simulink model "Modelo_NL_Final"  (R2018a)
settings: Solver=VariableStepAuto  StartTime=0.0  StopTime=2500  RelTol=1e-3
values from neighbouring files (symbols this model uses):
  A = [xu,        xw*u0,         -u0*tan(aa0), -g*cos(tt0),     0 ... (first row only)    [long_ctes.m]    (also in modelo_L13_PD_lateral.m = [ybb yp+w0/u0 yr-1 g*cos(tt0)/u0 ; lbb lp lr 0 ; nbb np nr 0; real_servo_c_lateral.m = [ybb yp+w0/u0 yr-1 g*cos(tt0)/u0 0; lbb lp lr 0 0; nbb np nr)
  A_lat = [ybb yp+w0/u0 yr-1 g*cos(tt0)/u0 0; lbb lp lr 0 0; nbb np nr 0 0; 0 1 tan(tt0) 0 0; 0 0 1/cos(tt0) 0 0]    [lateral_ctes.m]
  B = [xde,         xdf ... (first row only)    [long_ctes.m]    (also in modelo_L13_PD_lateral.m = [0 Ydr ; Lda Ldr ; Nda Ndr ; 0 0]; real_servo_c_lateral.m = [0 Ydr ; Lda Ldr ; Nda Ndr ; 0 0 ; 0 0])
  B_lat = [0 Ydr ; Lda Ldr ; Nda Ndr ; 0 0 ; 0 0]    [lateral_ctes.m]
  C_lat = eye(5)    [lateral_ctes.m]
  Cc_lat = C_lat(2:1:4,:)    [lateral_ctes.m]
  Cy_lat = C_lat(1:4:5,:)    [lateral_ctes.m]
  D_lat = [0 0; 0 0; 0 0; 0 0; 0 0]    [lateral_ctes.m]
  deg = pi/180    (= 0.0174532925199)    [lateral_ctes.m]    (also in long_ctes.m; modelo_L13_PD_lateral.m; real_servo_c_lateral.m)
  demax = 28*deg    (= 0.488692190558)    [long_ctes.m]    (also in modelo_L13_PD_lateral.m = [+28 -21]; real_servo_c_lateral.m = [+28 -21])
  demin = -21*deg    (= -0.366519142919)    [long_ctes.m]
  inicial = [u0, aa0, 0, tt0, h0]    [long_ctes.m]
  Kc = [-0.0196 1.6622 -0.8045 -3.0813 -0.0000 0.9333]    [long_ctes.m]    (also in real_servo_c_lateral.m = k(:,2:1:4))
  Kc_lat = k_lat(:,2:1:4)    [lateral_ctes.m]
  Ky_lat = k_lat(:,1:4:5)    [lateral_ctes.m]
  pontos_T = pontos.'    [coordenadas2.m]
libraries: simulink x7, dspsigops x1
settings Model: Creator=tiagogomes  LastModifiedBy=tiagogomes
settings DataIOCC: ReturnWorkspaceOutputs=on
settings SFSimCC: SimUseLocalCustomCode=on
settings RTWCC: RTWUseLocalCustomCode=on

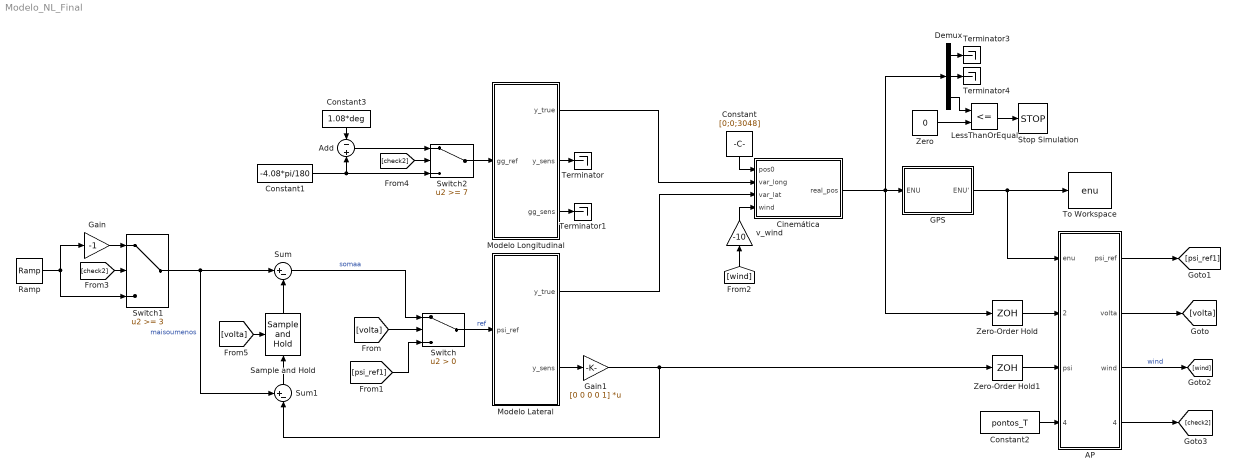
== system Modelo_NL_Final ==
  AP : MATLAB Function  TreatAsAtomicUnit=on
  Add : Sum  Inputs=-+
  Cinemática : Subsystem
  Constant : Constant  Value=[0;0;3048]
  Constant1 : Constant  Value=-4.08*pi/180
  Constant2 : Constant  Value=pontos_T
  Constant3 : Constant  Value=1.08*deg
  Demux : Demux  Outputs=3
  GPS : Subsystem
  Gain : Gain  Gain=-1
  Gain1 : Gain  Gain=[0 0 0 0 1]  Multiplication=Matrix(K*u)
  LessThanOrEqual : RelationalOperator  Operator=<=  OutDataTypeStr=boolean  RndMeth=Simplest
  Modelo Lateral : Subsystem
  Modelo Longitudinal : Subsystem  TreatAsAtomicUnit=on
  Ramp : simulink/Sources/Ramp  slope=-0.192  start=0  InitialOutput=0
  Sample and Hold : dspsigops/Sample and Hold  trig=Rising edge  initCond=0  latchinput=off
  Stop Simulation : Stop
  Sum : Sum  Inputs=|+-
  Sum1 : Sum  Inputs=+-|
  Switch : Switch  Criteria=u2 > Threshold
  Switch1 : Switch  Threshold=3
  Switch2 : Switch  Threshold=7
  Terminator{,1,3..4} (4 alike) : Terminator
  To Workspace : ToWorkspace  VariableName=enu  SampleTime=-1
      settings: Save2DSignal=2-D array (concatenate along first dimension)
  Zero : Constant  Value=0  OutDataTypeStr=Inherit: Inherit via back propagation
  Zero-Order Hold : ZeroOrderHold
  Zero-Order Hold1 : ZeroOrderHold
  v_wind : Gain  Gain=-10
  wires:
  Constant/1 -> Cinemática/1(pos0)
  Modelo Longitudinal/1(y_true) -> Cinemática/2(var_long)
  Modelo Lateral/1(y_true) -> Cinemática/3(var_lat)
  Constant1/1 -> Add/2, Switch2/3
  Modelo Longitudinal/2(y_sens) -> Terminator/1
  Modelo Longitudinal/3(gg_sens) -> Terminator1/1
  Cinemática/1(real_pos) -> Zero-Order Hold/1, Demux/1, GPS/1(ENU)
  GPS/1(ENU') -> AP/1(enu), To Workspace/1
  Constant2/1 -> AP/4(pontos_T)
  v_wind/1 -> Cinemática/4(wind)
  [volta] -> Switch/2
  AP/1(psi_ref) -> [psi_ref1]
  Switch/1 -> Modelo Lateral/1(psi_ref)  "ref"
  [psi_ref1] -> Switch/3
  Zero-Order Hold/1 -> AP/2(enu_real)
  AP/2(volta) -> [volta]
  AP/3(wind) -> [wind]  "wind"
  [wind] -> v_wind/1
  Gain/1 -> Switch1/1
  AP/4(check2) -> [check2]
  [check2] -> Switch1/2
  Zero/1 -> LessThanOrEqual/2
  Demux/3 -> LessThanOrEqual/1
  LessThanOrEqual/1 -> Stop Simulation/1
  Constant3/1 -> Add/1
  Switch2/1 -> Modelo Longitudinal/1(gg_ref)
  Add/1 -> Switch2/1
  [check2] -> Switch2/2
  Demux/1 -> Terminator3/1
  Demux/2 -> Terminator4/1
  [volta] -> Sample and Hold/Trigger
  Modelo Lateral/2(y_sens) -> Gain1/1
  Gain1/1 -> Sum1/2, Zero-Order Hold1/1
  Sample and Hold/1 -> Sum/2
  Ramp/1 -> Switch1/3, Gain/1
  Sum1/1 -> Sample and Hold/1
  Switch1/1 -> Sum1/1, Sum/1  "maisoumenos"
  Sum/1 -> Switch/1  "somaa"
  Zero-Order Hold1/1 -> AP/3(psi)

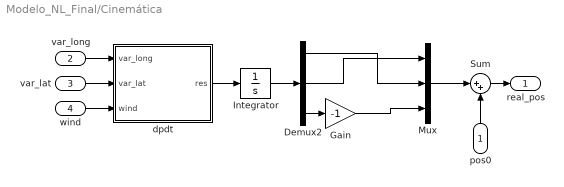
== system Modelo_NL_Final/Cinemática ==
  pos0 : Inport
  var_long : Inport  Port=2
  var_lat : Inport  Port=3
  wind : Inport  Port=4
  Demux2 : Demux  Outputs=3
  Gain : Gain  Gain=-1
  Integrator : Integrator
  Mux : Mux  Inputs=3
  Sum : Sum  Inputs=|++
  dpdt : MATLAB Function  TreatAsAtomicUnit=on
  real_pos : Outport
  wires:
  var_long/1 -> dpdt/1(var_long)
  wind/1 -> dpdt/3(wind)
  dpdt/1(res) -> Integrator/1
  Sum/1 -> real_pos/1
  var_lat/1 -> dpdt/2(var_lat)
  pos0/1 -> Sum/2
  Integrator/1 -> Demux2/1
  Demux2/1 -> Mux/2
  Mux/1 -> Sum/1
  Demux2/2 -> Mux/1
  Demux2/3 -> Gain/1
  Gain/1 -> Mux/3

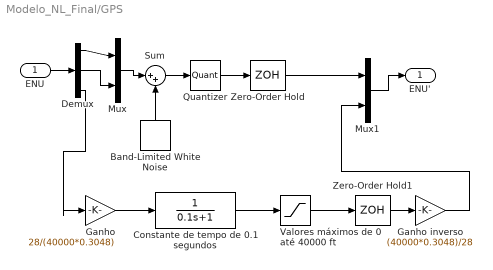
== system Modelo_NL_Final/GPS ==
  ENU : Inport
  Band-Limited White Noise : simulink/Sources/Band-Limited White Noise  Cov=16  Ts=1  seed=[23341]
  Constante de tempo de 0.1 segundos : TransferFcn  Denominator=[0.1 1]
  Demux : Demux  Outputs=3
  Ganho : Gain  Gain=28/(40000*0.3048)
  Ganho inverso : Gain  Gain=(40000*0.3048)/28
  Mux : Mux  Inputs=2
  Mux1 : Mux  Inputs=2
  Quantizer : Quantizer
  Sum : Sum  Inputs=|++
  Valores máximos de 0 até 40000 ft : Saturate  UpperLimit=28  LowerLimit=0
  Zero-Order Hold : ZeroOrderHold
  Zero-Order Hold1 : ZeroOrderHold
  ENU' : Outport
  wires:
  Sum/1 -> Quantizer/1
  Quantizer/1 -> Zero-Order Hold/1
  Band-Limited White Noise/1 -> Sum/2
  Ganho/1 -> Constante de tempo de 0.1 segundos/1
  Ganho inverso/1 -> Mux1/2
  Constante de tempo de 0.1 segundos/1 -> Valores máximos de 0 até 40000 ft/1
  ENU/1 -> Demux/1
  Demux/2 -> Mux/2
  Demux/1 -> Mux/1
  Mux/1 -> Sum/1
  Demux/3 -> Ganho/1
  Zero-Order Hold/1 -> Mux1/1
  Mux1/1 -> ENU'/1
  Valores máximos de 0 até 40000 ft/1 -> Zero-Order Hold1/1
  Zero-Order Hold1/1 -> Ganho inverso/1

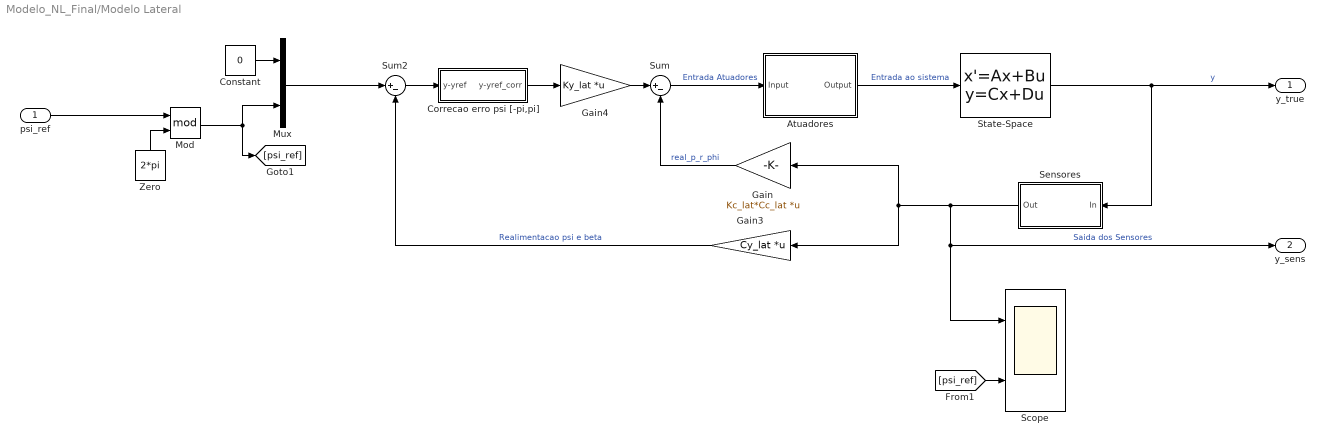
== system Modelo_NL_Final/Modelo Lateral ==
  psi_ref : Inport
  Atuadores : Subsystem
  Constant : Constant  Value=0
  Correcao erro psi [-pi,pi] : Subsystem
  Gain : Gain  Gain=Kc_lat*Cc_lat  Multiplication=Matrix(K*u)
  Gain3 : Gain  Gain=Cy_lat  Multiplication=Matrix(K*u)
  Gain4 : Gain  Gain=Ky_lat  Multiplication=Matrix(K*u)
  Mod : Math  Operator=mod  SaturateOnIntegerOverflow=on
  Mux : Mux  Inputs=2
  Scope : Scope  NumInputPorts=2
  Sensores : Subsystem
  State-Space : StateSpace  A=A_lat  B=B_lat  C=C_lat  D=D_lat  InitialCondition=[0 0 0 0 2.8254]  ContinuousStateAttributes={'beta','p','r','pranchamento','guinada'}
  Sum : Sum  Inputs=|+-
  Sum2 : Sum  Inputs=|+-
  Zero : Constant  Value=2*pi  OutDataTypeStr=Inherit: Inherit via back propagation
  y_true : Outport
  y_sens : Outport  Port=2
  wires:
  Constant/1 -> Mux/1
  Correcao erro psi [-pi,pi]/1(y-yref_corr) -> Gain4/1
  Mod/1 -> Mux/2, [psi_ref]
  State-Space/1 -> y_true/1, Sensores/1(In)  "y"
  Gain4/1 -> Sum/1
  Mux/1 -> Sum2/1
  Sensores/1(Out) -> Gain/1, Gain3/1, Scope/1, y_sens/1  "Saida dos Sensores"
  Gain/1 -> Sum/2  "real_p_r_phi"
  Atuadores/1(Output) -> State-Space/1  "Entrada ao sistema"
  [psi_ref] -> Scope/2
  Gain3/1 -> Sum2/2  "Realimentacao psi e beta"
  Sum/1 -> Atuadores/1(Input)  "Entrada Atuadores"
  Sum2/1 -> Correcao erro psi [-pi,pi]/1(y-yref)
  Zero/1 -> Mod/2
  psi_ref/1 -> Mod/1

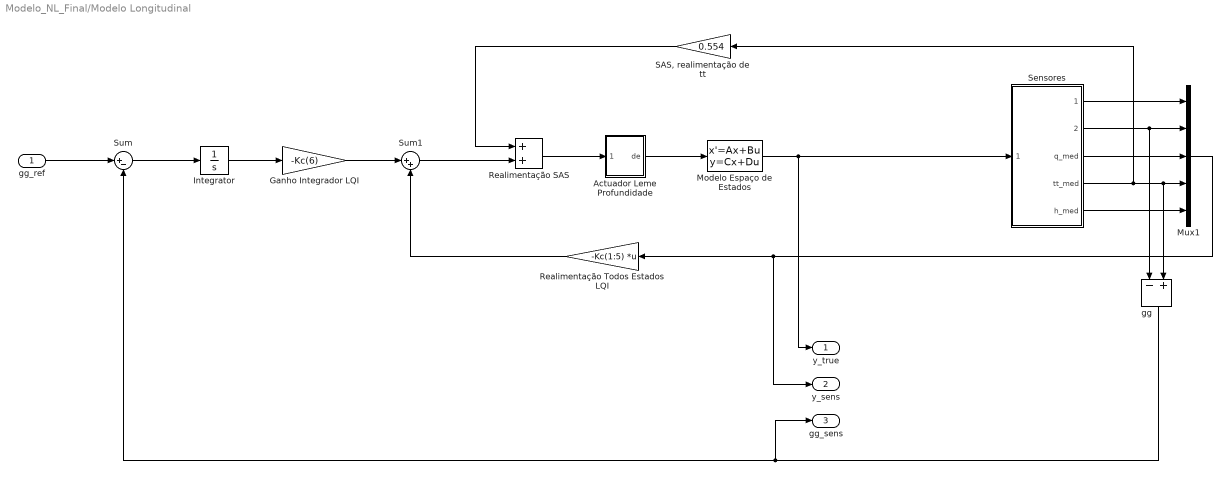
== system Modelo_NL_Final/Modelo Longitudinal ==
  gg_ref : Inport
  "Actuador Leme Profundidade " : Subsystem
  Ganho Integrador LQI : Gain  Gain=-Kc(6)
  Integrator : Integrator
  Modelo Espaço de Estados : StateSpace  A=A  B=B(:,1)  C=eye(5)  D=[0; 0; 0; 0; 0]  InitialCondition=inicial  ContinuousStateAttributes={'u', 'aa', 'q', 'tt', 'h'}
  Mux1 : Mux  Inputs=5
  Realimentação SAS : Sum
  Realimentação Todos Estados LQI : Gain  Gain=-Kc(1:5)  Multiplication=Matrix(K*u) (u vector)
  "SAS, realimentação de tt" : Gain  Gain=0.554
  Sensores : Subsystem
  Sum : Sum  Inputs=|+-
  Sum1 : Sum  Inputs=|++
  gg : Sum  Inputs=-+
  y_true : Outport
  y_sens : Outport  Port=2
  gg_sens : Outport  Port=3
  wires:
  gg_ref/1 -> Sum/1
  Sum/1 -> Integrator/1
  Integrator/1 -> Ganho Integrador LQI/1
  Ganho Integrador LQI/1 -> Sum1/1
  "Actuador Leme Profundidade "/1(de) -> Modelo Espaço de Estados/1
  "SAS, realimentação de tt"/1 -> Realimentação SAS/1
  Sum1/1 -> Realimentação SAS/2
  Realimentação Todos Estados LQI/1 -> Sum1/2
  Realimentação SAS/1 -> "Actuador Leme Profundidade "/1(de0)
  Modelo Espaço de Estados/1 -> Sensores/1(Estados), y_true/1
  Sensores/4(tt_med) -> gg/2, Mux1/4, "SAS, realimentação de tt"/1
  Sensores/1(TAS_med) -> Mux1/1
  Sensores/2(aa_med) -> gg/1, Mux1/2
  Sensores/3(q_med) -> Mux1/3
  Sensores/5(h_med) -> Mux1/5
  Mux1/1 -> y_sens/1, Realimentação Todos Estados LQI/1
  gg/1 -> gg_sens/1, Sum/2

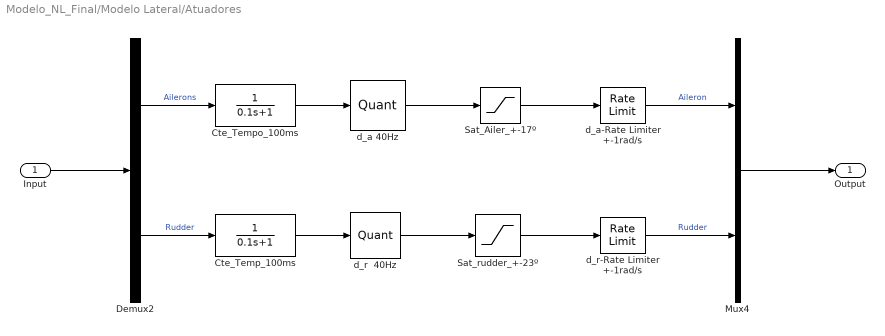
== system Modelo_NL_Final/Modelo Lateral/Atuadores ==
  Input : Inport
  Cte_Temp_100ms : TransferFcn  Denominator=[0.1 1]
  Cte_Tempo_100ms : TransferFcn  Denominator=[0.1 1]
  Demux2 : Demux  Outputs=2
  Mux4 : Mux  Inputs=2
  Sat_Ailer_+-17º : Saturate  UpperLimit=17*deg  LowerLimit=-17*deg
  Sat_rudder_+-23º : Saturate  UpperLimit=23*deg  LowerLimit=-23*deg
  d_a 40Hz : Quantizer  QuantizationInterval=1/40
  d_a-Rate Limiter +-1rad/s : RateLimiter  SampleTimeMode=inherited
  d_r  40Hz : Quantizer  QuantizationInterval=1/40
  d_r-Rate Limiter +-1rad/s : RateLimiter  SampleTimeMode=inherited
  Output : Outport
  wires:
  d_a 40Hz/1 -> Sat_Ailer_+-17º/1
  Input/1 -> Demux2/1
  Sat_rudder_+-23º/1 -> d_r-Rate Limiter +-1rad/s/1
  Mux4/1 -> Output/1
  Cte_Temp_100ms/1 -> d_r  40Hz/1
  d_r  40Hz/1 -> Sat_rudder_+-23º/1
  d_r-Rate Limiter +-1rad/s/1 -> Mux4/2  "Rudder"
  Demux2/2 -> Cte_Temp_100ms/1  "Rudder"
  d_a-Rate Limiter +-1rad/s/1 -> Mux4/1  "Aileron"
  Demux2/1 -> Cte_Tempo_100ms/1  "Ailerons"
  Cte_Tempo_100ms/1 -> d_a 40Hz/1
  Sat_Ailer_+-17º/1 -> d_a-Rate Limiter +-1rad/s/1

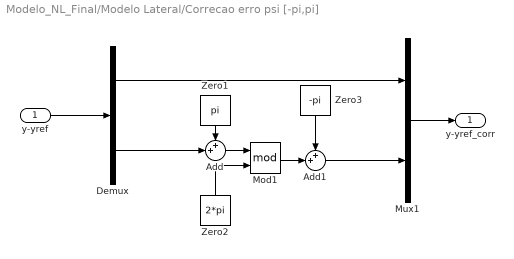
== system Modelo_NL_Final/Modelo Lateral/Correcao erro psi [-pi,pi] ==
  y-yref : Inport
  Add : Sum  Inputs=++|
  Add1 : Sum  Inputs=++|
  Demux : Demux  Outputs=2
  Mod1 : Math  Operator=mod  SaturateOnIntegerOverflow=on
  Mux1 : Mux  Inputs=2
  Zero1 : Constant  Value=pi  OutDataTypeStr=Inherit: Inherit via back propagation
  Zero2 : Constant  Value=2*pi  OutDataTypeStr=Inherit: Inherit via back propagation
  Zero3 : Constant  Value=-pi  OutDataTypeStr=Inherit: Inherit via back propagation
  y-yref_corr : Outport
  wires:
  Zero1/1 -> Add/1
  Zero3/1 -> Add1/1
  Zero2/1 -> Mod1/2
  Mod1/1 -> Add1/2
  y-yref/1 -> Demux/1
  Add/1 -> Mod1/1
  Mux1/1 -> y-yref_corr/1
  Add1/1 -> Mux1/2
  Demux/2 -> Add/2
  Demux/1 -> Mux1/1

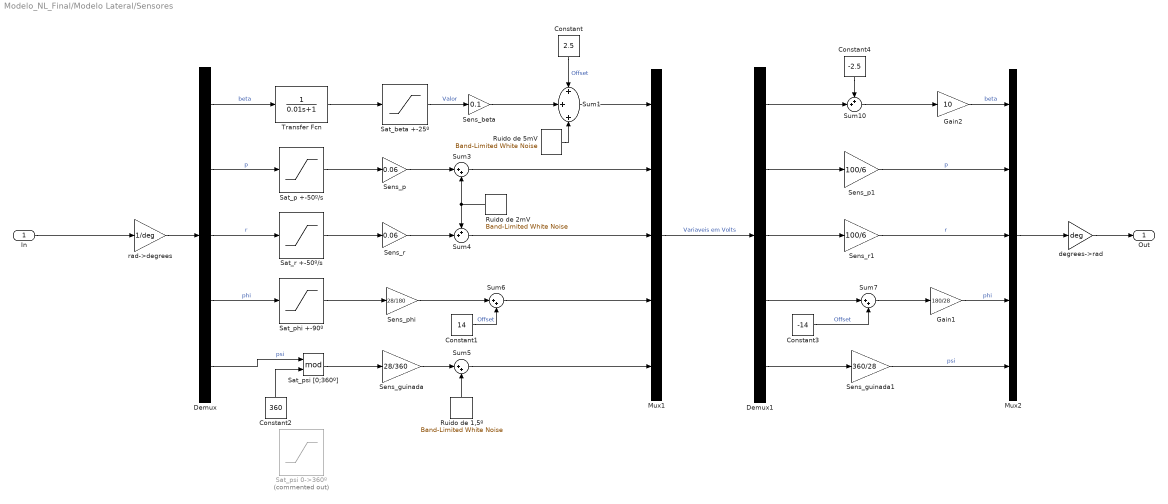
== system Modelo_NL_Final/Modelo Lateral/Sensores ==
  In : Inport
  Constant : Constant  Value=2.5
  Constant1 : Constant  Value=14
  Constant2 : Constant  Value=360
  Constant3 : Constant  Value=-14
  Constant4 : Constant  Value=-2.5
  Demux : Demux  Outputs=5
  Demux1 : Demux  Outputs=5
  Gain1 : Gain  Gain=180/28
  Gain2 : Gain  Gain=10
  Mux1 : Mux  Inputs=5
  Mux2 : Mux  Inputs=5
  Ruido de 1,5º : simulink/Sources/Band-Limited White Noise  Cov=[(1.5*28/360)^2/40]  Ts=1/40  seed=[23341]
  Ruido de 2mV : simulink/Sources/Band-Limited White Noise  Cov=[(0.002)^2/40]  Ts=1/40  seed=[23341]
  Ruido de 5mV : simulink/Sources/Band-Limited White Noise  Cov=[(0.005)^2/40]  Ts=1/40  seed=[23341]
  Sat_beta +-25º : Saturate  UpperLimit=+25  LowerLimit=-25
  Sat_p +-50º/s : Saturate  UpperLimit=+50  LowerLimit=-50
  Sat_phi +-90º : Saturate  UpperLimit=+90  LowerLimit=-90
  Sat_psi 0->360º : Saturate  Commented=on  UpperLimit=360  LowerLimit=-360
  Sat_psi [0;360º] : Math  Operator=mod  SaturateOnIntegerOverflow=on
  Sat_r +-50º/s : Saturate  UpperLimit=+50  LowerLimit=-50
  Sens_beta : Gain  Gain=0.1
  Sens_guinada : Gain  Gain=28/360
  Sens_guinada1 : Gain  Gain=360/28
  Sens_p : Gain  Gain=0.06
  Sens_p1 : Gain  Gain=100/6
  Sens_phi : Gain  Gain=28/180
  Sens_r : Gain  Gain=0.06
  Sens_r1 : Gain  Gain=100/6
  Sum1 : Sum  Inputs=+++
  Sum10 : Sum  Inputs=++|
  Sum{3,5..7} (4 alike) : Sum  Inputs=|++
  Sum4 : Sum  Inputs=++|
  Transfer Fcn : TransferFcn  Denominator=[0.01 1]
  degrees->rad : Gain  Gain=deg
  rad->degrees : Gain  Gain=1/deg
  Out : Outport
  wires:
  Sens_guinada/1 -> Sum5/1
  Demux1/4 -> Sum7/1
  Gain2/1 -> Mux2/1  "beta"
  Sens_phi/1 -> Sum6/1
  Demux1/5 -> Sens_guinada1/1
  Sat_p +-50º/s/1 -> Sens_p/1
  Sum6/1 -> Mux1/4
  Sens_p1/1 -> Mux2/2  "p"
  Constant1/1 -> Sum6/2  "Offset"
  Sens_beta/1 -> Sum1/2
  Ruido de 5mV/1 -> Sum1/3
  Sens_r1/1 -> Mux2/3  "r"
  In/1 -> rad->degrees/1
  Sat_beta +-25º/1 -> Sens_beta/1  "Valor"
  Constant3/1 -> Sum7/2  "Offset"
  degrees->rad/1 -> Out/1
  Sum4/1 -> Mux1/3
  Demux/4 -> Sat_phi +-90º/1  "phi"
  Sum7/1 -> Gain1/1
  Sens_r/1 -> Sum4/2
  Sum10/1 -> Gain2/1
  Gain1/1 -> Mux2/4  "phi"
  rad->degrees/1 -> Demux/1
  Mux1/1 -> Demux1/1  "Variaveis em Volts"
  Sens_guinada1/1 -> Mux2/5  "psi"
  Sum5/1 -> Mux1/5
  Sat_phi +-90º/1 -> Sens_phi/1
  Demux/2 -> Sat_p +-50º/s/1  "p"
  Sum1/1 -> Mux1/1
  Demux/3 -> Sat_r +-50º/s/1  "r"
  Ruido de 1,5º/1 -> Sum5/2
  Ruido de 2mV/1 -> Sum3/2, Sum4/1
  Mux2/1 -> degrees->rad/1
  Sens_p/1 -> Sum3/1
  Sum3/1 -> Mux1/2
  Constant/1 -> Sum1/1  "Offset"
  Sat_r +-50º/s/1 -> Sens_r/1
  Demux1/3 -> Sens_r1/1
  Demux1/2 -> Sens_p1/1
  Demux/1 -> Transfer Fcn/1  "beta"
  Transfer Fcn/1 -> Sat_beta +-25º/1
  Demux1/1 -> Sum10/2
  Constant4/1 -> Sum10/1
  Demux/5 -> Sat_psi [0;360º]/1  "psi"
  Sat_psi [0;360º]/1 -> Sens_guinada/1
  Constant2/1 -> Sat_psi [0;360º]/2

== system Modelo_NL_Final/Modelo Longitudinal/Actuador Leme Profundidade  ==
  de0 : Inport
  Amostragem 40Hz : ZeroOrderHold  SampleTime=1/40
  Constante de tempo de 0.1 segundos : TransferFcn  Denominator=[0.1 1]
  Deflexões máximas +28º / -21º : Saturate  UpperLimit=demax  LowerLimit=demin
  Velocidade deflexão máxima 1 rad/s : RateLimiter  SampleTimeMode=inherited
  de : Outport
  wires:
  de0/1 -> Constante de tempo de 0.1 segundos/1
  Constante de tempo de 0.1 segundos/1 -> Amostragem 40Hz/1
  Amostragem 40Hz/1 -> Deflexões máximas +28º / -21º/1
  Deflexões máximas +28º / -21º/1 -> Velocidade deflexão máxima 1 rad/s/1
  Velocidade deflexão máxima 1 rad/s/1 -> de/1

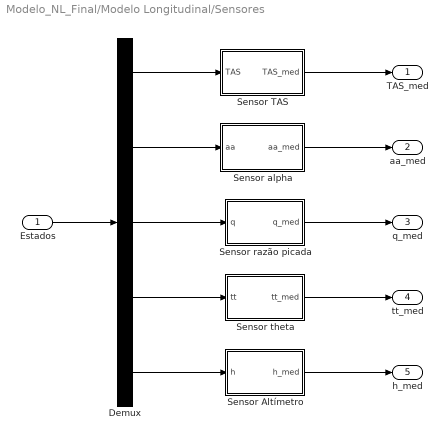
== system Modelo_NL_Final/Modelo Longitudinal/Sensores ==
  Estados : Inport
  Demux : Demux  Outputs=5
  "Sensor Altímetro " : Subsystem
  Sensor TAS : Subsystem
  Sensor alpha : Subsystem
  Sensor razão picada : Subsystem
  Sensor theta : Subsystem
  TAS_med : Outport
  aa_med : Outport  Port=2
  q_med : Outport  Port=3
  tt_med : Outport  Port=4
  h_med : Outport  Port=5
  wires:
  Estados/1 -> Demux/1
  Demux/1 -> Sensor TAS/1(TAS)
  Demux/2 -> Sensor alpha/1(aa)
  Demux/3 -> Sensor razão picada/1(q)
  Demux/4 -> Sensor theta/1(tt)
  Demux/5 -> "Sensor Altímetro "/1(h)
  Sensor TAS/1(TAS_med) -> TAS_med/1
  Sensor alpha/1(aa_med) -> aa_med/1
  Sensor razão picada/1(q_med) -> q_med/1
  Sensor theta/1(tt_med) -> tt_med/1
  "Sensor Altímetro "/1(h_med) -> h_med/1

== system Modelo_NL_Final/Modelo Longitudinal/Sensores/Sensor Altímetro  ==
  h : Inport
  Constante de tempo de 0.1 segundos : TransferFcn  Denominator=[0.1 1]
  Ganho : Gain  Gain=28/(40000*0.3048)
  Ganho inverso : Gain  Gain=(40000*0.3048)/28
  Valores máximos de 0 até 40000 ft : Saturate  UpperLimit=28  LowerLimit=0
  h_med : Outport
  wires:
  Constante de tempo de 0.1 segundos/1 -> Valores máximos de 0 até 40000 ft/1
  Valores máximos de 0 até 40000 ft/1 -> Ganho inverso/1
  h/1 -> Ganho/1
  Ganho/1 -> Constante de tempo de 0.1 segundos/1
  Ganho inverso/1 -> h_med/1

== system Modelo_NL_Final/Modelo Longitudinal/Sensores/Sensor TAS ==
  TAS : Inport
  Constante de tempo de 0.05 segundos : TransferFcn  Denominator=[0.05 1]
  Ganho : Gain  Gain=28/(1000*0.5144)
  Ganho Inverso : Gain  Gain=(1000*0.5144)/28
  Valores máximos de medição 0-1000 knt : Saturate  UpperLimit=28  LowerLimit=0
  TAS_med : Outport
  wires:
  Constante de tempo de 0.05 segundos/1 -> Valores máximos de medição 0-1000 knt/1
  Valores máximos de medição 0-1000 knt/1 -> Ganho Inverso/1
  TAS/1 -> Ganho/1
  Ganho/1 -> Constante de tempo de 0.05 segundos/1
  Ganho Inverso/1 -> TAS_med/1

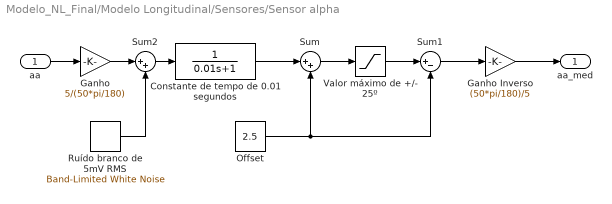
== system Modelo_NL_Final/Modelo Longitudinal/Sensores/Sensor alpha ==
  aa : Inport
  Constante de tempo de 0.01 segundos : TransferFcn  Denominator=[0.01 1]
  Ganho : Gain  Gain=5/(50*pi/180)
  Ganho Inverso : Gain  Gain=(50*pi/180)/5
  Offset : Constant  Value=2.5
  Ruído branco de 5mV RMS : simulink/Sources/Band-Limited White Noise  Cov=[0.000000625]  Ts=1/40  seed=[23341]  VectorParams1D=off
  Sum : Sum  Inputs=|++
  Sum1 : Sum  Inputs=|+-
  Sum2 : Sum  Inputs=|++
  Valor máximo de +/- 25º : Saturate  UpperLimit=5  LowerLimit=0
  aa_med : Outport
  wires:
  aa/1 -> Ganho/1
  Constante de tempo de 0.01 segundos/1 -> Sum/1
  Sum/1 -> Valor máximo de +/- 25º/1
  Valor máximo de +/- 25º/1 -> Sum1/1
  Offset/1 -> Sum1/2, Sum/2
  Sum1/1 -> Ganho Inverso/1
  Ganho Inverso/1 -> aa_med/1
  Ganho/1 -> Sum2/1
  Sum2/1 -> Constante de tempo de 0.01 segundos/1
  Ruído branco de 5mV RMS/1 -> Sum2/2

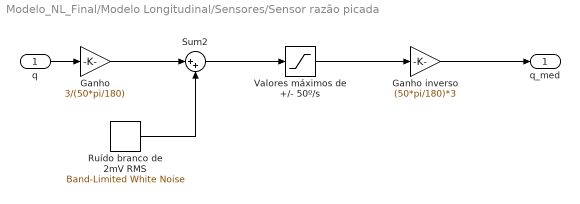
== system Modelo_NL_Final/Modelo Longitudinal/Sensores/Sensor razão picada ==
  q : Inport
  Ganho : Gain  Gain=3/(50*pi/180)
  Ganho inverso : Gain  Gain=(50*pi/180)*3
  Ruído branco de 2mV RMS : simulink/Sources/Band-Limited White Noise  Cov=[0.0000001]  Ts=1/40  seed=[23341]
  Sum2 : Sum  Inputs=|++
  Valores máximos de +/- 50º/s : Saturate  UpperLimit=3  LowerLimit=-3
  q_med : Outport
  wires:
  q/1 -> Ganho/1
  Ganho inverso/1 -> q_med/1
  Ganho/1 -> Sum2/1
  Ruído branco de 2mV RMS/1 -> Sum2/2
  Sum2/1 -> Valores máximos de +/- 50º/s/1
  Valores máximos de +/- 50º/s/1 -> Ganho inverso/1

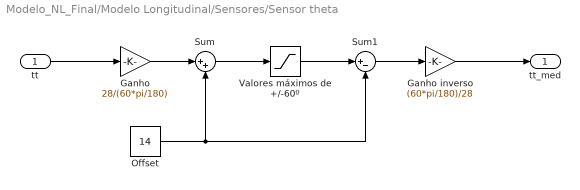
== system Modelo_NL_Final/Modelo Longitudinal/Sensores/Sensor theta ==
  tt : Inport
  Ganho : Gain  Gain=28/(60*pi/180)
  Ganho inverso : Gain  Gain=(60*pi/180)/28
  "Offset " : Constant  Value=14
  Sum : Sum  Inputs=|++
  Sum1 : Sum  Inputs=|+-
  Valores máximos de +/-60º : Saturate  UpperLimit=28  LowerLimit=0
  tt_med : Outport
  wires:
  Ganho inverso/1 -> tt_med/1
  tt/1 -> Ganho/1
  "Offset "/1 -> Sum/2, Sum1/2
  Ganho/1 -> Sum/1
  Sum/1 -> Valores máximos de +/-60º/1
  Valores máximos de +/-60º/1 -> Sum1/1
  Sum1/1 -> Ganho inverso/1

== matlab function Modelo_NL_Final/AP ==
  data: enu input; enu_real input; psi input; psi_ref output; volta output; pontos_T input; wind output; check2 output
function [psi_ref, volta, wind, check2] = way(enu, enu_real, psi, pontos_T)

    persistent check
    if isempty(check)
        check = 2;
    end
    
    persistent volta0
    if isempty(volta0)
        volta0 = 0;
    end
    
    r = pontos_T(:,check) - enu(1:2);
    r_real = pontos_T(:,check) - enu_real(1:2);
    
    if norm(r)>240
        d_psi = asin(190/norm(r));
    else
        d_psi = 0;
        if (check == 2 || check == 3)
            volta0 = 1;
        end
    end
    
    
    if check == 2
        psi_ref = pi/2 - atan2(r(2),r(1)) + d_psi; 
    elseif check == 3
        psi_ref = pi/2 - atan2(r(2),r(1)) - d_psi; 
    else
        psi_ref = pi/2 - atan2(r(2),r(1));
    end
    
    if norm(r_real)<200 && (check==2 || check==3)
        wind = 1;
    else
        wind = 0;
    end
    
    if norm(r) < 200 && check < 8
        r = pontos_T(:,check+1) - enu(1:2);
        psi_s = pi/2 - atan2(r(2),r(1));
        if (check == 2 && enu(3)>2500 && psi < psi_s+0.3 && psi > psi_s-0.3) || (check == 3 && enu(3) > 1700 && psi < psi_s+0.3 && psi > psi_s-0.3) || (check > 3)
            volta0 = 0;
            check = check + 1;
        end
    end
        
    volta = volta0;
    check2=check;
end

== matlab function Modelo_NL_Final/Cinemática/dpdt ==
  data: var_long input; res output; var_lat input; wind input
function res = dpdt(var_long,var_lat,wind)
    phi = var_lat(4);
    tt  = var_long(4);
    psi = var_lat(5);
    
    u = var_long(1);
    v = sin(var_lat(1))*u;
    w = tan(var_long(2))*u;
    
    S = [1 0 0; 0 cos(phi) sin(phi); 0 -sin(phi) cos(phi)]*[cos(tt) 0 -sin(tt); 0 1 0; sin(tt) 0 cos(tt)]*[cos(psi) sin(psi) 0; -sin(psi) cos(psi) 0; 0 0 1];
    
    v_a = [u;v;w];
    v_w = [0;0;wind];
    
    res = (S.')*v_a + v_w;
    
end
